simulink model "Excavator_Mevea_BucketDriveline"  (R2026a)
settings: Solver=ode23t  StopTime=29.5  FixedStep=1e-5  MaxStep=Ts  AbsTol=1e-3
PostLoadFcn:
  | set_param(bdroot,'IgnoredZcDiagnostic','none');
  | Excavator_Test_Scenario_Select('loadedBucketDigCycle');
  | Excavator_Mevea_params
StartFcn:
  | tic
StopFcn:
  | elapsedSimTime = toc;
  | disp(['Elapsed Sim Time = ' num2str(elapsedSimTime)]);
model workspace: external: MAT-File ExcavatorAssemblyDataStruct.mat (data not in the file)
undefined symbols (not defined in the file or in its folder): AToBRegOrificeVector, AToTOrificeVector, BiPOrificeVector, BoomC, boomHEArea, boomREArea, boomUpMaxQ, boomValve, BToTOrificeVector, BucketC, bucketCloseMaxQ, bucketOpenMaxQ, BucketR, bucketValve, DiscIntNeverNeededParam, fluids, gravity, K, Lambda, LeftBoomR, maxPumpDisp, minPumpDisp, nominalEngineSpeed, P28Assembly, PToAOrificeVector, PToBOrificeVector, pumpCmdNegRateLimit, pumpCmdPosRateLimit, RightBoomR, StickC, stickInMaxQ, stickOutMaxQ, StickR, stickValve, SwingC, swingDisplacement, swingHighSpeedThreshold, swingMaxQ, SwingR, swingSpeedQGain, swingValve, tau, valveCmdNegRateLimit, valveCmdPosRateLimit, X, x0, Y, Z
libraries: fl_lib x113, SimscapeFluids_lib x78, nesl_utility x61, sm_lib x55, simulink_extras x11, Excavator_Parts_Lib x6, sm_wheel_loader_lib x6, simulink x5, sdl_lib x4, SignalEditorBlockLib x1
(part 5 of 8)

== system Excavator_Mevea_BucketDriveline/Excavator/Machine/Boom Cyl R/BoomRightCyl ==
  BoomRightCyl_primary : sm_lib/Body Elements/File Solid  ExtGeomFileName=BoomRightCyl_Primary.SLDPRT  UnitType=FromFile  ExtGeomFileUnits=m  StepReaderType=HEX  ExportConvexHullGeometry=off  InertiaType=Custom  BasedOnType=DensityFromFile  Density=1000  DensityUnits=kg/m^3  Mass=P28Assembly.bodyGroups(4).subGroups(1).inertialProperties.mass  MassUnits=kg  CenterOfMass=P28Assembly.bodyGroups(4).subGroups(1).inertialProperties.centerOfMass  CenterOfMassUnits=m  MomentsOfInertia=P28Assembly.bodyGroups(4).subGroups(1).inertialProperties.momentsOfInertia  MomentsOfInertiaUnits=kg*m^2  ProductsOfInertia=P28Assembly.bodyGroups(4).subGroups(1).inertialProperties.productsOfInertia  ProductsOfInertiaUnits=kg*m^2  GraphicType=FromGeometry  MarkerShape=Sphere  MarkerSize=10  GraphicVisPropType=SimpleVisualProperties  GraphicDiffuseColor=P28Assembly.bodyGroups(4).subGroups(1).visualProperties.rgb  GraphicOpacity=P28Assembly.bodyGroups(4).subGroups(1).visualProperties.opacity  GraphicSpecularColor=[0.5 0.5 0.5 1.0]  GraphicAmbientColor=[0.15 0.15 0.15 1.0]  GraphicEmissiveColor=[0.0 0.0 0.0 1.0]  GraphicShininess=75  DoExposeReferenceFrame=on  SerializedFrames=<Frames/>
  RT_ChassisToRightBoomCyl : sm_lib/Frames and Transforms/Rigid Transform  RotationMethod=RotationMatrix  FollAlignAxisA=+X  BaseAlignAxisA=+Y  FollAlignAxisB=+Y  BaseAlignAxisB=+Z  RotationStandardAxis=+Z  RotationAngle=0.0  RotationAngleUnits=deg  RotationArbitraryAxis=[0 0 1]  RotationSequenceAxes=FollowerAxes  RotationSequence=XYX  RotationSequenceAngles=[0 0 0]  RotationSequenceAnglesUnits=deg  RotationMatrix=P28Assembly.coordSys(6).transform.rotation  Quaternion=[1 0 0 0]  TranslationMethod=Cartesian  TranslationCartesianOffset=P28Assembly.coordSys(6).transform.translation  TranslationCartesianOffsetUnits=m  TranslationStandardAxis=+Z  TranslationStandardOffset=0  TranslationStandardOffsetUnits=m  TranslationROffset=0  TranslationROffsetUnits=m  TranslationThetaOffset=0  TranslationThetaOffsetUnits=deg  TranslationZOffset=0  TranslationZOffsetUnits=m
  RT_RightBoomCylToRightBoomPiston : sm_lib/Frames and Transforms/Rigid Transform  RotationMethod=RotationMatrix  FollAlignAxisA=+X  BaseAlignAxisA=+Y  FollAlignAxisB=+Y  BaseAlignAxisB=+Z  RotationStandardAxis=+Z  RotationAngle=0.0  RotationAngleUnits=deg  RotationArbitraryAxis=[0 0 1]  RotationSequenceAxes=FollowerAxes  RotationSequence=XYX  RotationSequenceAngles=[0 0 0]  RotationSequenceAnglesUnits=deg  RotationMatrix=P28Assembly.coordSys(19).transform.rotation  Quaternion=[1 0 0 0]  TranslationMethod=Cartesian  TranslationCartesianOffset=P28Assembly.coordSys(19).transform.translation  TranslationCartesianOffsetUnits=m  TranslationStandardAxis=+Z  TranslationStandardOffset=0  TranslationStandardOffsetUnits=m  TranslationROffset=0  TranslationROffsetUnits=m  TranslationThetaOffset=0  TranslationThetaOffsetUnits=deg  TranslationZOffset=0  TranslationZOffsetUnits=m
  B1 : PMIOPort  Side=Left
  F1 : PMIOPort  Port=2  Side=Right
  connections:
  RT_RightBoomCylToRightBoomPiston/RConn1 -- F1/RConn1
  RT_ChassisToRightBoomCyl/RConn1 -- B1/RConn1
  RT_RightBoomCylToRightBoomPiston/LConn1 -- BoomRightCyl_primary/RConn1 -- RT_ChassisToRightBoomCyl/LConn1

== system Excavator_Mevea_BucketDriveline/Excavator/Machine/Boom Cyl R/BoomRightPiston ==
  BoomRightPiston_primary : sm_lib/Body Elements/File Solid  ExtGeomFileName=BoomRightPiston_Primary.SLDPRT  UnitType=FromFile  ExtGeomFileUnits=m  StepReaderType=HEX  ExportConvexHullGeometry=off  InertiaType=Custom  BasedOnType=DensityFromFile  Density=1000  DensityUnits=kg/m^3  Mass=P28Assembly.bodyGroups(5).subGroups(1).inertialProperties.mass  MassUnits=kg  CenterOfMass=P28Assembly.bodyGroups(5).subGroups(1).inertialProperties.centerOfMass  CenterOfMassUnits=m  MomentsOfInertia=P28Assembly.bodyGroups(5).subGroups(1).inertialProperties.momentsOfInertia  MomentsOfInertiaUnits=kg*m^2  ProductsOfInertia=P28Assembly.bodyGroups(5).subGroups(1).inertialProperties.productsOfInertia  ProductsOfInertiaUnits=kg*m^2  GraphicType=FromGeometry  MarkerShape=Sphere  MarkerSize=10  GraphicVisPropType=SimpleVisualProperties  GraphicDiffuseColor=P28Assembly.bodyGroups(5).subGroups(1).visualProperties.rgb  GraphicOpacity=P28Assembly.bodyGroups(5).subGroups(1).visualProperties.opacity  GraphicSpecularColor=[0.5 0.5 0.5 1.0]  GraphicAmbientColor=[0.15 0.15 0.15 1.0]  GraphicEmissiveColor=[0.0 0.0 0.0 1.0]  GraphicShininess=75  DoExposeReferenceFrame=on  SerializedFrames=<Frames/>
  RT_BoomToRightBoomPiston : sm_lib/Frames and Transforms/Rigid Transform  RotationMethod=RotationMatrix  FollAlignAxisA=+X  BaseAlignAxisA=+Y  FollAlignAxisB=+Y  BaseAlignAxisB=+Z  RotationStandardAxis=+Z  RotationAngle=0.0  RotationAngleUnits=deg  RotationArbitraryAxis=[0 0 1]  RotationSequenceAxes=FollowerAxes  RotationSequence=XYX  RotationSequenceAngles=[0 0 0]  RotationSequenceAnglesUnits=deg  RotationMatrix=P28Assembly.coordSys(7).transform.rotation  Quaternion=[1 0 0 0]  TranslationMethod=Cartesian  TranslationCartesianOffset=P28Assembly.coordSys(7).transform.translation  TranslationCartesianOffsetUnits=m  TranslationStandardAxis=+Z  TranslationStandardOffset=0  TranslationStandardOffsetUnits=m  TranslationROffset=0  TranslationROffsetUnits=m  TranslationThetaOffset=0  TranslationThetaOffsetUnits=deg  TranslationZOffset=0  TranslationZOffsetUnits=m
  RT_RightBoomCylToRightBoomPiston : sm_lib/Frames and Transforms/Rigid Transform  RotationMethod=RotationMatrix  FollAlignAxisA=+X  BaseAlignAxisA=+Y  FollAlignAxisB=+Y  BaseAlignAxisB=+Z  RotationStandardAxis=+Z  RotationAngle=0.0  RotationAngleUnits=deg  RotationArbitraryAxis=[0 0 1]  RotationSequenceAxes=FollowerAxes  RotationSequence=XYX  RotationSequenceAngles=[0 0 0]  RotationSequenceAnglesUnits=deg  RotationMatrix=P28Assembly.coordSys(19).transform.rotation  Quaternion=[1 0 0 0]  TranslationMethod=Cartesian  TranslationCartesianOffset=P28Assembly.coordSys(19).transform.translation  TranslationCartesianOffsetUnits=m  TranslationStandardAxis=+Z  TranslationStandardOffset=0  TranslationStandardOffsetUnits=m  TranslationROffset=0  TranslationROffsetUnits=m  TranslationThetaOffset=0  TranslationThetaOffsetUnits=deg  TranslationZOffset=0  TranslationZOffsetUnits=m
  B1 : PMIOPort  Side=Right
  B2 : PMIOPort  Port=2  Side=Left
  connections:
  RT_RightBoomCylToRightBoomPiston/RConn1 -- B2/RConn1
  RT_BoomToRightBoomPiston/RConn1 -- B1/RConn1
  RT_RightBoomCylToRightBoomPiston/LConn1 -- BoomRightPiston_primary/RConn1 -- RT_BoomToRightBoomPiston/LConn1

== system Excavator_Mevea_BucketDriveline/Excavator/Machine/Boom Cyl R/RightBoomCylToRightBoomPiston ==
  RightBoomCylToRightBoomPiston : sm_lib/Joints/Cylindrical Joint  JointMode=Normal  CompositeWrenchDir=FollowerOnBase  CompositeWrenchFrame=BaseFrame  SenseConstraintForce=off  SenseConstraintTorque=off  SenseTotalForce=off  SenseTotalTorque=off  RzPositionTargetSpecify=off  RzPositionTargetPriority=High  RzPositionTargetValue=0  RzPositionTargetValueUnits=deg  RzVelocityTargetSpecify=off  RzVelocityTargetPriority=High  RzVelocityTargetValue=0  RzVelocityTargetValueUnits=deg/s  RzEquilibriumPosition=0  RzEquilibriumPositionUnits=deg  RzSpringStiffness=0  RzSpringStiffnessUnits=N*m/deg  RzDampingCoefficient=0  RzDampingCoefficientUnits=N*m/(deg/s)  RzLowerLimitSpecify=off  RzLowerLimitBound=-90  RzLowerLimitBoundUnits=deg  RzLowerLimitStiffness=1e4  RzLowerLimitStiffnessUnits=N*m/deg  RzLowerLimitDamping=10  RzLowerLimitDampingUnits=N*m/(deg/s)  RzLowerLimitTransitionRegionWidth=0.1  RzLowerLimitTransitionRegionWidthUnits=deg  RzUpperLimitSpecify=off  RzUpperLimitBound=90  RzUpperLimitBoundUnits=deg  RzUpperLimitStiffness=1e4  RzUpperLimitStiffnessUnits=N*m/deg  RzUpperLimitDamping=10  RzUpperLimitDampingUnits=N*m/(deg/s)  RzUpperLimitTransitionRegionWidth=0.1  RzUpperLimitTransitionRegionWidthUnits=deg  RzTorqueActuationMode=NoTorque  RzMotionActuationMode=ComputedMotion  RzSensePosition=off  RzSenseVelocity=off  RzSenseAcceleration=off  RzSenseTorqueForce=off  RzSenseLowerLimitTorqueForce=off  RzSenseUpperLimitTorqueForce=off  PzPositionTargetSpecify=on  PzPositionTargetPriority=High  PzPositionTargetValue=initBoomPistonPos  PzPositionTargetValueUnits=mm  PzVelocityTargetSpecify=off  PzVelocityTargetPriority=High  PzVelocityTargetValue=0  PzVelocityTargetValueUnits=m/s  PzEquilibriumPosition=0  PzEquilibriumPositionUnits=m  PzSpringStiffness=0  PzSpringStiffnessUnits=N/m  PzDampingCoefficient=0  PzDampingCoefficientUnits=N/(m/s)  PzLowerLimitSpecify=off  PzLowerLimitBound=-1  PzLowerLimitBoundUnits=m  PzLowerLimitStiffness=1e6  PzLowerLimitStiffnessUnits=N/m  PzLowerLimitDamping=1e3  PzLowerLimitDampingUnits=N/(m/s)  PzLowerLimitTransitionRegionWidth=1e-4  PzLowerLimitTransitionRegionWidthUnits=m  PzUpperLimitSpecify=off  PzUpperLimitBound=1  PzUpperLimitBoundUnits=m  PzUpperLimitStiffness=1e6  PzUpperLimitStiffnessUnits=N/m  PzUpperLimitDamping=1e3  PzUpperLimitDampingUnits=N/(m/s)  PzUpperLimitTransitionRegionWidth=1e-4  PzUpperLimitTransitionRegionWidthUnits=m  PzTorqueActuationMode=InputTorque  PzMotionActuationMode=ComputedMotion  PzSensePosition=off  PzSenseVelocity=on  PzSenseAcceleration=off  PzSenseTorqueForce=off  PzSenseLowerLimitTorqueForce=off  PzSenseUpperLimitTorqueForce=off
  Simscape Bus : SimscapeBus  HierarchyStrings=BoomC;RightBoomR
  Translational Multibody Interface : fl_lib/Mechanical/Multibody Interfaces/Translational Multibody Interface
  BoomHydToMech : PMIOPort  Side=Left
  B : PMIOPort  Port=2  Side=Left
  F : PMIOPort  Port=3  Side=Right
  connections:
  RightBoomCylToRightBoomPiston/RConn1 -- F/RConn1
  RightBoomCylToRightBoomPiston/LConn1 -- B/RConn1
  Translational Multibody Interface/LConn1 -- RightBoomCylToRightBoomPiston/LConn2
  Translational Multibody Interface/RConn1 -- RightBoomCylToRightBoomPiston/RConn2
  Simscape Bus/RConn1 -- BoomHydToMech/RConn1
  Simscape Bus/LConn1 -- Translational Multibody Interface/LConn2
  Simscape Bus/LConn2 -- Translational Multibody Interface/RConn2

== system Excavator_Mevea_BucketDriveline/Excavator/Machine/Bucket Cyl/BucketCyl ==
  BucketCyl_primary : sm_lib/Body Elements/File Solid  ExtGeomFileName=BucketCyl_Primary.SLDPRT  UnitType=FromFile  ExtGeomFileUnits=m  StepReaderType=HEX  ExportConvexHullGeometry=off  InertiaType=Custom  BasedOnType=DensityFromFile  Density=1000  DensityUnits=kg/m^3  Mass=P28Assembly.bodyGroups(10).subGroups(1).inertialProperties.mass  MassUnits=kg  CenterOfMass=P28Assembly.bodyGroups(10).subGroups(1).inertialProperties.centerOfMass  CenterOfMassUnits=m  MomentsOfInertia=P28Assembly.bodyGroups(10).subGroups(1).inertialProperties.momentsOfInertia  MomentsOfInertiaUnits=kg*m^2  ProductsOfInertia=P28Assembly.bodyGroups(10).subGroups(1).inertialProperties.productsOfInertia  ProductsOfInertiaUnits=kg*m^2  GraphicType=FromGeometry  MarkerShape=Sphere  MarkerSize=10  GraphicVisPropType=SimpleVisualProperties  GraphicDiffuseColor=P28Assembly.bodyGroups(10).subGroups(1).visualProperties.rgb  GraphicOpacity=P28Assembly.bodyGroups(10).subGroups(1).visualProperties.opacity  GraphicSpecularColor=[0.5 0.5 0.5 1.0]  GraphicAmbientColor=[0.15 0.15 0.15 1.0]  GraphicEmissiveColor=[0.0 0.0 0.0 1.0]  GraphicShininess=75  DoExposeReferenceFrame=on  SerializedFrames=<Frames/>
  RT_BucketCylToBucketPiston : sm_lib/Frames and Transforms/Rigid Transform  RotationMethod=RotationMatrix  FollAlignAxisA=+X  BaseAlignAxisA=+Y  FollAlignAxisB=+Y  BaseAlignAxisB=+Z  RotationStandardAxis=+Z  RotationAngle=0.0  RotationAngleUnits=deg  RotationArbitraryAxis=[0 0 1]  RotationSequenceAxes=FollowerAxes  RotationSequence=XYX  RotationSequenceAngles=[0 0 0]  RotationSequenceAnglesUnits=deg  RotationMatrix=P28Assembly.coordSys(21).transform.rotation  Quaternion=[1 0 0 0]  TranslationMethod=Cartesian  TranslationCartesianOffset=P28Assembly.coordSys(21).transform.translation  TranslationCartesianOffsetUnits=m  TranslationStandardAxis=+Z  TranslationStandardOffset=0  TranslationStandardOffsetUnits=m  TranslationROffset=0  TranslationROffsetUnits=m  TranslationThetaOffset=0  TranslationThetaOffsetUnits=deg  TranslationZOffset=0  TranslationZOffsetUnits=m
  RT_StickToBucketCyl : sm_lib/Frames and Transforms/Rigid Transform  RotationMethod=RotationMatrix  FollAlignAxisA=+X  BaseAlignAxisA=+Y  FollAlignAxisB=+Y  BaseAlignAxisB=+Z  RotationStandardAxis=+Z  RotationAngle=0.0  RotationAngleUnits=deg  RotationArbitraryAxis=[0 0 1]  RotationSequenceAxes=FollowerAxes  RotationSequence=XYX  RotationSequenceAngles=[0 0 0]  RotationSequenceAnglesUnits=deg  RotationMatrix=P28Assembly.coordSys(11).transform.rotation  Quaternion=[1 0 0 0]  TranslationMethod=Cartesian  TranslationCartesianOffset=P28Assembly.coordSys(11).transform.translation  TranslationCartesianOffsetUnits=m  TranslationStandardAxis=+Z  TranslationStandardOffset=0  TranslationStandardOffsetUnits=m  TranslationROffset=0  TranslationROffsetUnits=m  TranslationThetaOffset=0  TranslationThetaOffsetUnits=deg  TranslationZOffset=0  TranslationZOffsetUnits=m
  B1 : PMIOPort  Side=Left
  F1 : PMIOPort  Port=2  Side=Right
  connections:
  RT_StickToBucketCyl/LConn1 -- BucketCyl_primary/RConn1 -- RT_BucketCylToBucketPiston/LConn1
  RT_StickToBucketCyl/RConn1 -- B1/RConn1
  RT_BucketCylToBucketPiston/RConn1 -- F1/RConn1

== system Excavator_Mevea_BucketDriveline/Excavator/Machine/Bucket Cyl/BucketCylToBucketPiston ==
  BucketCylToBucketPiston : sm_lib/Joints/Cylindrical Joint  JointMode=Normal  CompositeWrenchDir=FollowerOnBase  CompositeWrenchFrame=BaseFrame  SenseConstraintForce=off  SenseConstraintTorque=off  SenseTotalForce=off  SenseTotalTorque=off  RzPositionTargetSpecify=off  RzPositionTargetPriority=High  RzPositionTargetValue=0  RzPositionTargetValueUnits=deg  RzVelocityTargetSpecify=off  RzVelocityTargetPriority=High  RzVelocityTargetValue=0  RzVelocityTargetValueUnits=deg/s  RzEquilibriumPosition=0  RzEquilibriumPositionUnits=deg  RzSpringStiffness=0  RzSpringStiffnessUnits=N*m/deg  RzDampingCoefficient=0  RzDampingCoefficientUnits=N*m/(deg/s)  RzLowerLimitSpecify=off  RzLowerLimitBound=-90  RzLowerLimitBoundUnits=deg  RzLowerLimitStiffness=1e4  RzLowerLimitStiffnessUnits=N*m/deg  RzLowerLimitDamping=10  RzLowerLimitDampingUnits=N*m/(deg/s)  RzLowerLimitTransitionRegionWidth=0.1  RzLowerLimitTransitionRegionWidthUnits=deg  RzUpperLimitSpecify=off  RzUpperLimitBound=90  RzUpperLimitBoundUnits=deg  RzUpperLimitStiffness=1e4  RzUpperLimitStiffnessUnits=N*m/deg  RzUpperLimitDamping=10  RzUpperLimitDampingUnits=N*m/(deg/s)  RzUpperLimitTransitionRegionWidth=0.1  RzUpperLimitTransitionRegionWidthUnits=deg  RzTorqueActuationMode=NoTorque  RzMotionActuationMode=ComputedMotion  RzSensePosition=off  RzSenseVelocity=off  RzSenseAcceleration=off  RzSenseTorqueForce=off  RzSenseLowerLimitTorqueForce=off  RzSenseUpperLimitTorqueForce=off  PzPositionTargetSpecify=on  PzPositionTargetPriority=High  PzPositionTargetValue=initBucketPistonPos  PzPositionTargetValueUnits=mm  PzVelocityTargetSpecify=off  PzVelocityTargetPriority=High  PzVelocityTargetValue=0  PzVelocityTargetValueUnits=m/s  PzEquilibriumPosition=0  PzEquilibriumPositionUnits=m  PzSpringStiffness=0  PzSpringStiffnessUnits=N/m  PzDampingCoefficient=0  PzDampingCoefficientUnits=N/(m/s)  PzLowerLimitSpecify=off  PzLowerLimitBound=-1  PzLowerLimitBoundUnits=m  PzLowerLimitStiffness=1e6  PzLowerLimitStiffnessUnits=N/m  PzLowerLimitDamping=1e3  PzLowerLimitDampingUnits=N/(m/s)  PzLowerLimitTransitionRegionWidth=1e-4  PzLowerLimitTransitionRegionWidthUnits=m  PzUpperLimitSpecify=off  PzUpperLimitBound=1  PzUpperLimitBoundUnits=m  PzUpperLimitStiffness=1e6  PzUpperLimitStiffnessUnits=N/m  PzUpperLimitDamping=1e3  PzUpperLimitDampingUnits=N/(m/s)  PzUpperLimitTransitionRegionWidth=1e-4  PzUpperLimitTransitionRegionWidthUnits=m  PzTorqueActuationMode=InputTorque  PzMotionActuationMode=ComputedMotion  PzSensePosition=off  PzSenseVelocity=on  PzSenseAcceleration=off  PzSenseTorqueForce=off  PzSenseLowerLimitTorqueForce=off  PzSenseUpperLimitTorqueForce=off
  Simscape Bus : SimscapeBus  HierarchyStrings=BucketC;BucketR
  Translational Multibody Interface : fl_lib/Mechanical/Multibody Interfaces/Translational Multibody Interface
  B : PMIOPort  Side=Left
  F : PMIOPort  Port=2  Side=Right
  BucketHydToMech : PMIOPort  Port=3  Side=Left
  connections:
  B/RConn1 -- BucketCylToBucketPiston/LConn1
  Simscape Bus/RConn1 -- BucketHydToMech/RConn1
  Translational Multibody Interface/LConn2 -- Simscape Bus/LConn1
  Simscape Bus/LConn2 -- Translational Multibody Interface/RConn2
  Translational Multibody Interface/RConn1 -- BucketCylToBucketPiston/RConn2
  Translational Multibody Interface/LConn1 -- BucketCylToBucketPiston/LConn2
  BucketCylToBucketPiston/RConn1 -- F/RConn1

== system Excavator_Mevea_BucketDriveline/Excavator/Machine/Bucket Cyl/BucketPiston ==
  BucketPiston_primary : sm_lib/Body Elements/File Solid  ExtGeomFileName=BucketPiston_Primary.SLDPRT  UnitType=FromFile  ExtGeomFileUnits=m  StepReaderType=HEX  ExportConvexHullGeometry=off  InertiaType=Custom  BasedOnType=DensityFromFile  Density=1000  DensityUnits=kg/m^3  Mass=P28Assembly.bodyGroups(11).subGroups(1).inertialProperties.mass  MassUnits=kg  CenterOfMass=P28Assembly.bodyGroups(11).subGroups(1).inertialProperties.centerOfMass  CenterOfMassUnits=m  MomentsOfInertia=P28Assembly.bodyGroups(11).subGroups(1).inertialProperties.momentsOfInertia  MomentsOfInertiaUnits=kg*m^2  ProductsOfInertia=P28Assembly.bodyGroups(11).subGroups(1).inertialProperties.productsOfInertia  ProductsOfInertiaUnits=kg*m^2  GraphicType=FromGeometry  MarkerShape=Sphere  MarkerSize=10  GraphicVisPropType=SimpleVisualProperties  GraphicDiffuseColor=P28Assembly.bodyGroups(11).subGroups(1).visualProperties.rgb  GraphicOpacity=P28Assembly.bodyGroups(11).subGroups(1).visualProperties.opacity  GraphicSpecularColor=[0.5 0.5 0.5 1.0]  GraphicAmbientColor=[0.15 0.15 0.15 1.0]  GraphicEmissiveColor=[0.0 0.0 0.0 1.0]  GraphicShininess=75  DoExposeReferenceFrame=on  SerializedFrames=<Frames/>
  RT_BucketCylToBucketPiston : sm_lib/Frames and Transforms/Rigid Transform  RotationMethod=RotationMatrix  FollAlignAxisA=+X  BaseAlignAxisA=+Y  FollAlignAxisB=+Y  BaseAlignAxisB=+Z  RotationStandardAxis=+Z  RotationAngle=0.0  RotationAngleUnits=deg  RotationArbitraryAxis=[0 0 1]  RotationSequenceAxes=FollowerAxes  RotationSequence=XYX  RotationSequenceAngles=[0 0 0]  RotationSequenceAnglesUnits=deg  RotationMatrix=P28Assembly.coordSys(21).transform.rotation  Quaternion=[1 0 0 0]  TranslationMethod=Cartesian  TranslationCartesianOffset=P28Assembly.coordSys(21).transform.translation  TranslationCartesianOffsetUnits=m  TranslationStandardAxis=+Z  TranslationStandardOffset=0  TranslationStandardOffsetUnits=m  TranslationROffset=0  TranslationROffsetUnits=m  TranslationThetaOffset=0  TranslationThetaOffsetUnits=deg  TranslationZOffset=0  TranslationZOffsetUnits=m
  RT_BucketPistonToBucketLink : sm_lib/Frames and Transforms/Rigid Transform  RotationMethod=RotationMatrix  FollAlignAxisA=+X  BaseAlignAxisA=+Y  FollAlignAxisB=+Y  BaseAlignAxisB=+Z  RotationStandardAxis=+Z  RotationAngle=0.0  RotationAngleUnits=deg  RotationArbitraryAxis=[0 0 1]  RotationSequenceAxes=FollowerAxes  RotationSequence=XYX  RotationSequenceAngles=[0 0 0]  RotationSequenceAnglesUnits=deg  RotationMatrix=P28Assembly.coordSys(12).transform.rotation  Quaternion=[1 0 0 0]  TranslationMethod=Cartesian  TranslationCartesianOffset=P28Assembly.coordSys(12).transform.translation  TranslationCartesianOffsetUnits=m  TranslationStandardAxis=+Z  TranslationStandardOffset=0  TranslationStandardOffsetUnits=m  TranslationROffset=0  TranslationROffsetUnits=m  TranslationThetaOffset=0  TranslationThetaOffsetUnits=deg  TranslationZOffset=0  TranslationZOffsetUnits=m
  B1 : PMIOPort  Side=Left
  F1 : PMIOPort  Port=2  Side=Right
  connections:
  BucketPiston_primary/RConn1 -- RT_BucketCylToBucketPiston/LConn1 -- RT_BucketPistonToBucketLink/LConn1
  RT_BucketCylToBucketPiston/RConn1 -- B1/RConn1
  RT_BucketPistonToBucketLink/RConn1 -- F1/RConn1

== system Excavator_Mevea_BucketDriveline/Excavator/Machine/Mevea/FMU ==
  mBucket : Inport
  mChassis : Inport  Port=2
  mRight : Inport  Port=3
  mLeft : Inport  Port=4
  Brk : Inport  Port=5
  Demux : Demux  Outputs=13
  Demux11 : Demux  Outputs=13
  FMU : FMU  FMUName=MeveaLargeExcavatorTCFMUCSControl.fmu  FMUMode=CoSimulation  FMUInitializeEnumObject=off  FMUCachedDialogLayout="{\"Geometry\":[2658,147,869,770],\"ParameterColumnsWidthConfig\":\"{\\\"columns\\\":[{\\\"name\\\":\\\"Parameter\\\",\\\"width\\\":223},{\\\"name\\\":\\\"Value\\\",\\\"width\\\":194},{\\\"name\\\":\\\"Unit\\\",\\\"width\\\":186},{\\\"name\\\":\\\"Description\\\",\\\"width\\\":229}]}\",\"InputColumnsWidthConfig\":\"{\\\"columns\\\":[{\\\"name\\\":\\\"Name\\\",\\\"width\\\":189},{\\\"name\\\":\\\"Visibility\\\",\\\"width\\\":60},{\\\"name\\\":\\\"Start\\\",\\\"width\\\":181},{\\\"name\\\":\\\"Unit\\\",\\\"width\\\":177},{\\\"name\\\":\\\"Type Object\\\",\\\"width\\\":221}]}\",\"OutputColumnsWidthConfig\":[]}"  DV_RollerHeigth=-0.73  DV_RollerDistance=0.35  DV_Roller1_Posx=2.1  DV_Roller2_Posx=1.75  DV_Roller3_Posx=1.4  DV_Roller4_Posx=1.05  DV_Roller5_Posx=0.7  DV_Roller6_Posx=0.35  DV_Roller7_Posx=0  DV_Roller8_Posx=-0.35  DV_Roller9_Posx=-0.70  DV_Roller10_Posx=-1.05  DV_Roller11_Posx=-1.4  DV_Roller12_Posx=-1.75  DV_Roller13_Posx=-2.1  DV_SprocketRadius=0.50  DV_RollerRadius=0.15  DV_RollerDamping=3  DV_SprocketDamping=5  DV_SprocketMass=615  socketPort=int32(5111)  useHeadlessSolver=int32(0)  activateAssemblies="\"\""  deactivateAssemblies="\"\""  solverIPaddress='127.0.0.1'  mask(MeveaExcavatorExternalCSControl [Co-Simulation, v2.0]){}
      mask Display:
      | disp('MeveaExcavatorExternalCSControl');
      | port_label('output',1,'SO_BucketForce_X');
      | port_label('output',2,'SO_BucketForce_Y');
      | port_label('output',3,'SO_BucketForce_Z');
      | port_label('output',4,'SO_BucketTorque_X');
      | port_label('output',5,'SO_BucketTorque_Y');
      | port_label('output',6,'SO_BucketTorque_Z');
      | port_label('output',7,'SO_UndercarriageForce_X');
      | port_label('output',8,'SO_UndercarriageForce_Y');
      | port_label('output',9,'SO_UndercarriageForce_Z');
      | port_label('output',10,'SO_UndercarriageTorque_X');
      | port_label('output',11,'SO_UndercarriageTorque_Y');
      | port_label('output',12,'SO_UndercarriageTorque_Z');
      | port_label('output',13,'SO_LeftCrawler_w');
      | port_label('output',14,'SO_RightCrawler_w');
      | port_label('input',1,'SI_BucketVelocity_X');
      | port_label('input',2,'SI_BucketVelocity_Y');
      | port_label('input',3,'SI_BucketVelocity_Z');
      | port_label('input',4,'SI_BucketOmega_X');
      | port_label('input',5,'SI_BucketOmega_Y');
      | port_label('input',6,'SI_BucketOmega_Z');
      | port_label('input',7,'SI_BucketPosition_X');
      | port_label('input',8,'SI_BucketPosition_Y');
      | port_label('input',9,'SI_BucketPosition_Z');
      | port_label('input',10,'SI_BucketQuat_w');
      | port_label('input',11,'SI_BucketQuat_ux');
      | port_label('input',12,'SI_BucketQuat_uy');
      | port_label('input',13,'SI_BucketQuat_uz');
      | port_label('input',14,'SI_UndercarriageVelocity_X');
      | port_label('input',15,'SI_UndercarriageVelocity_Y');
      | port_label('input',16,'SI_UndercarriageVelocity_Z');
      | port_label('input',17,'SI_UndercarriageOmega_X');
      | port_label('input',18,'SI_UndercarriageOmega_Y');
      | port_label('input',19,'SI_UndercarriageOmega_Z');
      | port_label('input',20,'SI_UndercarriagePosition_X');
      | port_label('input',21,'SI_UndercarriagePosition_Y');
      | port_label('input',22,'SI_UndercarriagePosition_Z');
      | port_label('input',23,'SI_UndercarriageQuat_w');
      | port_label('input',24,'SI_UndercarriageQuat_ux');
      | port_label('input',25,'SI_UndercarriageQuat_uy');
      | port_label('input',26,'SI_UndercarriageQuat_uz');
      | port_label('input',27,'SI_LeftCrawler_T');
      | port_label('input',28,'SI_RightCrawler_T');
      | port_label('input',29,'SI_CrawlerBrake');
  Mux5 : Mux  Inputs=6
  Mux6 : Mux  Inputs=6
  fBucket : Outport
  fChassis : Outport  Port=2
  tRight : Outport  Port=3
  tLeft : Outport  Port=4
  wires:
  mChassis/1 -> Demux11/1
  Demux11/13 -> FMU/26
  FMU/10 -> Mux5/4
  Demux/2 -> FMU/2
  Brk/1 -> FMU/29
  FMU/13 -> tRight/1
  Demux11/12 -> FMU/25
  Demux/1 -> FMU/1
  FMU/8 -> Mux5/2
  Demux11/10 -> FMU/23
  FMU/4 -> Mux6/4
  Demux/9 -> FMU/9
  Demux11/11 -> FMU/24
  Demux/5 -> FMU/5
  FMU/2 -> Mux6/2
  Demux11/7 -> FMU/20
  FMU/5 -> Mux6/5
  Demux/6 -> FMU/6
  FMU/3 -> Mux6/3
  Demux/8 -> FMU/8
  Demux11/1 -> FMU/14
  FMU/9 -> Mux5/3
  FMU/7 -> Mux5/1
  Demux11/5 -> FMU/18
  Demux11/2 -> FMU/15
  Demux11/3 -> FMU/16
  Demux/13 -> FMU/13
  Demux11/6 -> FMU/19
  Demux11/4 -> FMU/17
  FMU/1 -> Mux6/1
  Demux11/8 -> FMU/21
  mLeft/1 -> FMU/27
  mRight/1 -> FMU/28
  Demux11/9 -> FMU/22
  Demux/10 -> FMU/10
  FMU/12 -> Mux5/6
  FMU/6 -> Mux6/6
  FMU/11 -> Mux5/5
  FMU/14 -> tLeft/1
  Demux/11 -> FMU/11
  Demux/12 -> FMU/12
  Demux/7 -> FMU/7
  Demux/4 -> FMU/4
  Demux/3 -> FMU/3
  Mux6/1 -> fBucket/1
  mBucket/1 -> Demux/1
  Mux5/1 -> fChassis/1

== system Excavator_Mevea_BucketDriveline/Excavator/Machine/Mevea/Forces Bucket ==
  ft : Inport
  Demux10 : Demux  Outputs=6
  First Order Hold : FirstOrderHold  ErrorTolerance=inf  AllowContinuousInput=on
  First Order Hold1 : FirstOrderHold  ErrorTolerance=inf  AllowContinuousInput=on
  Mux : Mux  Inputs=3
  Mux1 : Mux  Inputs=3
  Simulink-PS Converter2 : nesl_utility/Simulink-PS Converter  PhysicalDomain=network_engine_domain  SubClassName=ps_input  LeftPortType=input  RightPortType=output  PseudoPeriodic=off  Frequencies=[]  NoiseDistribution=none  NoiseParameters=[]  Unit=N  AffineConversion=off  FilteringAndDerivatives=provide  SimscapeFilterOrder=1  InputFilterTimeConstant=0.001  UdotUserProvided=0
  Simulink-PS Converter3 : nesl_utility/Simulink-PS Converter  PhysicalDomain=network_engine_domain  SubClassName=ps_input  LeftPortType=input  RightPortType=output  PseudoPeriodic=off  Frequencies=[]  NoiseDistribution=none  NoiseParameters=[]  Unit=N*m  AffineConversion=off  FilteringAndDerivatives=provide  SimscapeFilterOrder=1  InputFilterTimeConstant=0.001  UdotUserProvided=0
  frc : PMIOPort  Side=Right
  trq : PMIOPort  Port=2  Side=Right
  wires:
  Mux/1 -> First Order Hold/1
  Demux10/3 -> Mux/3
  First Order Hold1/1 -> Simulink-PS Converter3/1
  Demux10/6 -> Mux1/3
  Demux10/2 -> Mux/2
  Demux10/5 -> Mux1/2
  Mux1/1 -> First Order Hold1/1
  First Order Hold/1 -> Simulink-PS Converter2/1
  Demux10/1 -> Mux/1
  Demux10/4 -> Mux1/1
  ft/1 -> Demux10/1
  connections:
  Simulink-PS Converter2/RConn1 -- frc/RConn1
  Simulink-PS Converter3/RConn1 -- trq/RConn1

== system Excavator_Mevea_BucketDriveline/Excavator/Machine/Mevea/Forces Chassis ==
  ft : Inport
  Demux9 : Demux  Outputs=6
  First Order Hold2 : FirstOrderHold  ErrorTolerance=inf  AllowContinuousInput=on
  First Order Hold3 : FirstOrderHold  ErrorTolerance=inf  AllowContinuousInput=on
  Mux2 : Mux  Inputs=3
  Mux3 : Mux  Inputs=3
  Simulink-PS Converter1 : nesl_utility/Simulink-PS Converter  PhysicalDomain=network_engine_domain  SubClassName=ps_input  LeftPortType=input  RightPortType=output  PseudoPeriodic=off  Frequencies=[]  NoiseDistribution=none  NoiseParameters=[]  Unit=N  AffineConversion=off  FilteringAndDerivatives=provide  SimscapeFilterOrder=1  InputFilterTimeConstant=0.001  UdotUserProvided=0
  Simulink-PS Converter4 : nesl_utility/Simulink-PS Converter  PhysicalDomain=network_engine_domain  SubClassName=ps_input  LeftPortType=input  RightPortType=output  PseudoPeriodic=off  Frequencies=[]  NoiseDistribution=none  NoiseParameters=[]  Unit=N*m  AffineConversion=off  FilteringAndDerivatives=provide  SimscapeFilterOrder=1  InputFilterTimeConstant=0.001  UdotUserProvided=0
  frc : PMIOPort  Side=Right
  trq : PMIOPort  Port=2  Side=Right
  wires:
  Demux9/3 -> Mux2/3
  Demux9/6 -> Mux3/3
  Mux3/1 -> First Order Hold3/1
  Demux9/4 -> Mux3/1
  ft/1 -> Demux9/1
  Demux9/2 -> Mux2/2
  Mux2/1 -> First Order Hold2/1
  First Order Hold2/1 -> Simulink-PS Converter1/1
  Demux9/1 -> Mux2/1
  First Order Hold3/1 -> Simulink-PS Converter4/1
  Demux9/5 -> Mux3/2
  connections:
  Simulink-PS Converter4/RConn1 -- trq/RConn1
  Simulink-PS Converter1/RConn1 -- frc/RConn1

== system Excavator_Mevea_BucketDriveline/Excavator/Machine/Mevea/Interface CrawlerL ==
  note: Uncomment rate transition
      | blocks if one or both networks
      | are running fixed step.
  spd : Inport
  First Order Hold3 : FirstOrderHold  ErrorTolerance=inf  AllowContinuousInput=on
  Gain : Gain
  Gain1 : Gain  Gain=-1
  Ideal Rotational Motion Sensor : fl_lib/Mechanical/Mechanical Sensors/Ideal Rotational Motion Sensor  reference=foundation.enum.MeasurementReference.absolute  acceleration_port=false  velocity_port=true  position_port=false  wrap_angle=false  offset=0 rad
  Mux : Mux  Inputs=2
  PS-Simulink Converter : nesl_utility/PS-Simulink Converter  PhysicalDomain=network_engine_domain  SubClassName=ps_output  LeftPortType=input  RightPortType=output  PseudoPeriodic=off  Frequencies=[]  VectorFormat=inherit  Unit=rad/s  AffineConversion=off
  Port 1 Interface : Subsystem  mask(Network Coupler (Flexible Shaft) Port 1 Interface){interfaceModel=an actual shaft compliance, k=2500, lambda=200, samplingType=Variable step at ports 1 and 2, ts=0.002, h1=0.001, h2=0.01, predictionDiscreteToContinuous=off, smoothingContinuousToDiscrete=off, predictionSlowToFast=off, smoothingFastToSlow=off, nSmooth=1, tsSmoothing=0.01, J1=1, J2=1, tsRecommended=NaN, hRecommended=2.7764e-05, kDerived=2500, lambdaDerived=200, tsMax=0.012494, through0=0}
      mask prompts: interfaceModel "physmod:simscape:couplers:SimscapeNetworkCouplersLib:SeparateUsing_MP"; k "physmod:simscape:couplers:SimscapeNetworkCouplersLib:ShaftStiffnessNmrad_MP"; lambda "physmod:simscape:couplers:SimscapeNetworkCouplersLib:ShaftDampingNmrads_MP"; samplingType "physmod:simscape:couplers:SimscapeNetworkCouplersLib:SamplingType_MP"; ts "physmod:simscape:couplers:SimscapeNetworkCouplersLib:SeparatorTimeConstants_MP"; h1 "physmod:simscape:couplers:SimscapeNetworkCouplersLib:Port1NetworkDiscreteSampleTimes_MP"; h2 "physmod:simscape:couplers:SimscapeNetworkCouplersLib:Port2NetworkDiscreteSampleTimes_MP"; predictionDiscreteToContinuous "physmod:simscape:couplers:SimscapeNetworkCouplersLib:UsePredictionWhenConnectingFixedStepToVariableStep_MP"; smoothingContinuousToDiscrete "physmod:simscape:couplers:SimscapeNetworkCouplersLib:UseSmoothingWhenConnectingVariableStepToFixedStep_MP"; predictionSlowToFast "physmod:simscape:couplers:SimscapeNetworkCouplersLib:UsePredictionWhenConnectingSlowToFastSampleTimes_MP"; smoothingFastToSlow "physmod:simscape:couplers:SimscapeNetworkCouplersLib:UseSmoothingWhenConnectingFastToSlowSampleTimes_MP"; nSmooth "physmod:simscape:couplers:SimscapeNetworkCouplersLib:NumberOfSamplesOverWhichToSmooth_MP"; tsSmoothing "physmod:simscape:couplers:SimscapeNetworkCouplersLib:SmoothingTimeConstants_MP"; J1 "physmod:simscape:couplers:SimscapeNetworkCouplersLib:ApproximateInertiaAtPort1kgm2_MP"; J2 "physmod:simscape:couplers:SimscapeNetworkCouplersLib:ApproximateInertiaAtPort2kgm2_MP"; tsRecommended "physmod:simscape:couplers:SimscapeNetworkCouplersLib:RecommendedMaxFilterTimeConstants_MP"; hRecommended "physmod:simscape:couplers:SimscapeNetworkCouplersLib:RecommendedMaxDiscreteSampleTimes_MP"; kDerived "physmod:simscape:couplers:SimscapeNetworkCouplersLib:CalculatedShaftStiffnessNmrad_MP"; lambdaDerived "physmod:simscape:couplers:SimscapeNetworkCouplersLib:CalculatedShaftDampingNmrads_MP"; tsMax "physmod:simscape:couplers:SimscapeNetworkCouplersLib:CalculatedFastestTrackableTimeConstants_MP"; through0 "physmod:simscape:couplers:SimscapeNetworkCouplersLib:InitialTransmittedTorqueNm_MP"
      mask help: physmod:simscape:couplers:SimscapeNetworkCouplersLib:NetworkCouplerFlexibleShaftPort1Interface_MD
      mask init:
      | % Fixed step sample time value check
      | foundation.internal.couplers.checkSampleTimes(gcb,h1,h2);
      | 
      | % Map mask choices to Simscape block parameters  
      | [K,Lambda,tau,~,~,x0,~] = foundation.internal.couplers.mechanical.derivedParamsRotational(...
      |     gcb,ts,h1,h2,through0,k,lambda,J1,J2);
      settings: PortSchema="{\"entries\":[{\"content\":{\"sides\":[{\"content\":{\"connectorIds\":[\"LConn1\"]},\"type\":\"ConnectorPlacement.EquallySpacedRectSide\",\"uuid\":\"a6d4a9fd-b5aa-40dc-ab7e-2b646b9b57bc\"},{\"content\":{\"connectorIds\":[\"Out1\",\"In1\"],\"side\":\"RIGHT\"},\"type\":\"ConnectorPlacement.EquallySpacedRectSide\",\"uuid\":\"31bb6273-5b9b-48d0-a1a2-6fbacb979b97\"},{\"content\":{\"connectorIds\":[],\"side\":\"TOP\"},\"type\":\"ConnectorPlacement.EquallySpacedRectSide\",\"uuid\":\"0f7afab2-4481-486c-9ad0-2b42c5b091a4\"}]},\"type\":\"ConnectorPlacement.EquallySpacedConnector\",\"uuid\":\"a98e47aa-cbfd-441a-b14c-c9ea515c056e\"}],\"packageUris\":[\"http://schema.mathworks.com/mf0/Connector/R2020b\"],\"version\":\"1.0\"}"
      mask Help: web([docroot '/simscape/ref/networkcouplerflexibleshaft.html'])
      mask TypeOptions interfaceModel: physmod:simscape:couplers:SimscapeNetworkCouplersLib:anActualShaftCompliance_PV | physmod:simscape:couplers:SimscapeNetworkCouplersLib:anAddedNumericalCompliance_PV
      mask Callback interfaceModel: foundation.internal.couplers.mechanical.parameterVisibilities(gcb)
      mask TypeOptions samplingType: physmod:simscape:couplers:SimscapeNetworkCouplersLib:VariableStepAtPorts1And2_PV | physmod:simscape:couplers:SimscapeNetworkCouplersLib:VariableStepAtPort1AndFixedStepAtPort2_PV | physmod:simscape:couplers:SimscapeNetworkCouplersLib:FixedStepBothPortsWithCommonSampleTime_PV | physmod:simscape:couplers:SimscapeNetworkCouplersLib:FixedStepBothPortsWithFasterSamplingAtPort1_PV
      mask Callback samplingType: foundation.internal.couplers.mechanical.parameterVisibilities(gcb)
      mask Callback predictionDiscreteToContinuous: foundation.internal.couplers.mechanical.parameterVisibilities(gcb)
      mask Callback smoothingContinuousToDiscrete: foundation.internal.couplers.mechanical.parameterVisibilities(gcb)
      mask Callback predictionSlowToFast: foundation.internal.couplers.mechanical.parameterVisibilities(gcb)
      mask Callback smoothingFastToSlow: foundation.internal.couplers.mechanical.parameterVisibilities(gcb)
      mask DialogControl Main Prompt: physmod:simscape:couplers:SimscapeNetworkCouplersLib:tab_Main
      mask DialogControl interfaceModel Prompt: Separate using
      mask DialogControl k Prompt: Shaft stiffness (Nm/rad)
      mask DialogControl lambda Prompt: Shaft damping (Nm/(rad/s))
      mask DialogControl samplingType Prompt: Sampling type
      mask DialogControl ts Prompt: Separator time constant (s)
      mask DialogControl h1 Prompt: Port 1 network discrete sample time (s)
      mask DialogControl h2 Prompt: Port 2 network discrete sample time (s)
      mask DialogControl predictionDiscreteToContinuous Prompt: Use prediction when connecting fixed step to variable step
      mask DialogControl smoothingContinuousToDiscrete Prompt: Use smoothing when connecting variable step to fixed step
      mask DialogControl predictionSlowToFast Prompt: Use prediction when connecting slow to fast sample times
      mask DialogControl smoothingFastToSlow Prompt: Use smoothing when connecting fast to slow sample times
      mask DialogControl nSmooth Prompt: Number of samples over which to smooth
      mask DialogControl tsSmoothing Prompt: Smoothing time constant (s)
      mask DialogControl Analysis Prompt: physmod:simscape:couplers:SimscapeNetworkCouplersLib:tab_Analysis
      mask DialogControl connectedNetworkInfo Prompt: physmod:simscape:couplers:SimscapeNetworkCouplersLib:heading_ConnectedNetworkInformation
      mask DialogControl J1 Prompt: Approximate inertia at port 1 (kg*m^2)
      mask DialogControl J2 Prompt: Approximate inertia at port 2 (kg*m^2)
      mask DialogControl derivedValues Prompt: physmod:simscape:couplers:SimscapeNetworkCouplersLib:heading_DerivedValues
      mask DialogControl tsRecommended Prompt: Recommended max filter time constant (s)
      mask DialogControl hRecommended Prompt: Recommended max discrete sample time (s)
      mask DialogControl kDerived Prompt: Calculated shaft stiffness (Nm/rad)
      mask DialogControl lambdaDerived Prompt: Calculated shaft damping (Nm/(rad/s))
      mask DialogControl tsMax Prompt: Calculated fastest trackable time constant (s)
      mask DialogControl updateRecommendations Prompt: physmod:simscape:couplers:SimscapeNetworkCouplersLib:button_Update
      mask DialogControl updateRecommendations Callback: foundation.internal.couplers.mechanical.analysisRotational(gcb);
      mask DialogControl InitialConditions Prompt: physmod:simscape:couplers:SimscapeNetworkCouplersLib:tab_InitialConditions
      mask DialogControl through0 Prompt: Initial transmitted torque (Nm)
  Rate transition (fast-to-slow) : RateTransition  Integrity=off  OutPortSampleTime=mbsTimeStep
  Scope : Scope  NumInputPorts=2
      settings: ActiveDisplayYMinimum=-4.84019  ActiveDisplayYMaximum=4.44418
  E : PMIOPort  Side=Left
  trq : Outport
  wires:
  First Order Hold3/1 -> Gain/1
  Port 1 Interface/1(torque) -> Gain1/1
  PS-Simulink Converter/1 -> Mux/1
  Mux/1 -> Scope/1
  Rate transition (fast-to-slow)/1 -> Scope/2, trq/1
  spd/1 -> First Order Hold3/1, Mux/2
  Gain/1 -> Port 1 Interface/1(speed)
  Gain1/1 -> Rate transition (fast-to-slow)/1
  connections:
  E/RConn1 -- Ideal Rotational Motion Sensor/LConn1 -- Port 1 Interface/LConn1
  PS-Simulink Converter/LConn1 -- Ideal Rotational Motion Sensor/RConn1

== system Excavator_Mevea_BucketDriveline/Excavator/Machine/Mevea/Interface CrawlerR ==
  note: Uncomment rate transition
      | blocks if one or both networks
      | are running fixed step.
  spd : Inport
  First Order Hold3 : FirstOrderHold  ErrorTolerance=inf  AllowContinuousInput=on
  Gain : Gain
  Gain1 : Gain  Gain=-1
  Ideal Rotational Motion Sensor : fl_lib/Mechanical/Mechanical Sensors/Ideal Rotational Motion Sensor  reference=foundation.enum.MeasurementReference.absolute  acceleration_port=false  velocity_port=true  position_port=false  wrap_angle=false  offset=0 rad
  Mux : Mux  Inputs=2
  PS-Simulink Converter : nesl_utility/PS-Simulink Converter  PhysicalDomain=network_engine_domain  SubClassName=ps_output  LeftPortType=input  RightPortType=output  PseudoPeriodic=off  Frequencies=[]  VectorFormat=inherit  Unit=rad/s  AffineConversion=off
  Port 1 Interface : Subsystem  mask(Network Coupler (Flexible Shaft) Port 1 Interface){interfaceModel=an actual shaft compliance, k=2500, lambda=200, samplingType=Variable step at ports 1 and 2, ts=0.002, h1=0.001, h2=0.01, predictionDiscreteToContinuous=off, smoothingContinuousToDiscrete=off, predictionSlowToFast=off, smoothingFastToSlow=off, nSmooth=1, tsSmoothing=0.01, J1=1, J2=1, tsRecommended=NaN, hRecommended=2.7764e-05, kDerived=2500, lambdaDerived=200, tsMax=0.012494, through0=0}
      mask prompts: interfaceModel "physmod:simscape:couplers:SimscapeNetworkCouplersLib:SeparateUsing_MP"; k "physmod:simscape:couplers:SimscapeNetworkCouplersLib:ShaftStiffnessNmrad_MP"; lambda "physmod:simscape:couplers:SimscapeNetworkCouplersLib:ShaftDampingNmrads_MP"; samplingType "physmod:simscape:couplers:SimscapeNetworkCouplersLib:SamplingType_MP"; ts "physmod:simscape:couplers:SimscapeNetworkCouplersLib:SeparatorTimeConstants_MP"; h1 "physmod:simscape:couplers:SimscapeNetworkCouplersLib:Port1NetworkDiscreteSampleTimes_MP"; h2 "physmod:simscape:couplers:SimscapeNetworkCouplersLib:Port2NetworkDiscreteSampleTimes_MP"; predictionDiscreteToContinuous "physmod:simscape:couplers:SimscapeNetworkCouplersLib:UsePredictionWhenConnectingFixedStepToVariableStep_MP"; smoothingContinuousToDiscrete "physmod:simscape:couplers:SimscapeNetworkCouplersLib:UseSmoothingWhenConnectingVariableStepToFixedStep_MP"; predictionSlowToFast "physmod:simscape:couplers:SimscapeNetworkCouplersLib:UsePredictionWhenConnectingSlowToFastSampleTimes_MP"; smoothingFastToSlow "physmod:simscape:couplers:SimscapeNetworkCouplersLib:UseSmoothingWhenConnectingFastToSlowSampleTimes_MP"; nSmooth "physmod:simscape:couplers:SimscapeNetworkCouplersLib:NumberOfSamplesOverWhichToSmooth_MP"; tsSmoothing "physmod:simscape:couplers:SimscapeNetworkCouplersLib:SmoothingTimeConstants_MP"; J1 "physmod:simscape:couplers:SimscapeNetworkCouplersLib:ApproximateInertiaAtPort1kgm2_MP"; J2 "physmod:simscape:couplers:SimscapeNetworkCouplersLib:ApproximateInertiaAtPort2kgm2_MP"; tsRecommended "physmod:simscape:couplers:SimscapeNetworkCouplersLib:RecommendedMaxFilterTimeConstants_MP"; hRecommended "physmod:simscape:couplers:SimscapeNetworkCouplersLib:RecommendedMaxDiscreteSampleTimes_MP"; kDerived "physmod:simscape:couplers:SimscapeNetworkCouplersLib:CalculatedShaftStiffnessNmrad_MP"; lambdaDerived "physmod:simscape:couplers:SimscapeNetworkCouplersLib:CalculatedShaftDampingNmrads_MP"; tsMax "physmod:simscape:couplers:SimscapeNetworkCouplersLib:CalculatedFastestTrackableTimeConstants_MP"; through0 "physmod:simscape:couplers:SimscapeNetworkCouplersLib:InitialTransmittedTorqueNm_MP"
      mask help: physmod:simscape:couplers:SimscapeNetworkCouplersLib:NetworkCouplerFlexibleShaftPort1Interface_MD
      mask init: same as Excavator_Mevea_BucketDriveline/Excavator/Machine/Mevea/Interface CrawlerL/Port 1 Interface
      settings: PortSchema="{\"entries\":[{\"content\":{\"sides\":[{\"content\":{\"connectorIds\":[\"LConn1\"]},\"type\":\"ConnectorPlacement.EquallySpacedRectSide\",\"uuid\":\"a6d4a9fd-b5aa-40dc-ab7e-2b646b9b57bc\"},{\"content\":{\"connectorIds\":[\"Out1\",\"In1\"],\"side\":\"RIGHT\"},\"type\":\"ConnectorPlacement.EquallySpacedRectSide\",\"uuid\":\"31bb6273-5b9b-48d0-a1a2-6fbacb979b97\"},{\"content\":{\"connectorIds\":[],\"side\":\"TOP\"},\"type\":\"ConnectorPlacement.EquallySpacedRectSide\",\"uuid\":\"0f7afab2-4481-486c-9ad0-2b42c5b091a4\"}]},\"type\":\"ConnectorPlacement.EquallySpacedConnector\",\"uuid\":\"a98e47aa-cbfd-441a-b14c-c9ea515c056e\"}],\"packageUris\":[\"http://schema.mathworks.com/mf0/Connector/R2020b\"],\"version\":\"1.0\"}"
      mask Help: web([docroot '/simscape/ref/networkcouplerflexibleshaft.html'])
      mask TypeOptions interfaceModel: physmod:simscape:couplers:SimscapeNetworkCouplersLib:anActualShaftCompliance_PV | physmod:simscape:couplers:SimscapeNetworkCouplersLib:anAddedNumericalCompliance_PV
      mask Callback interfaceModel: foundation.internal.couplers.mechanical.parameterVisibilities(gcb)
      mask TypeOptions samplingType: physmod:simscape:couplers:SimscapeNetworkCouplersLib:VariableStepAtPorts1And2_PV | physmod:simscape:couplers:SimscapeNetworkCouplersLib:VariableStepAtPort1AndFixedStepAtPort2_PV | physmod:simscape:couplers:SimscapeNetworkCouplersLib:FixedStepBothPortsWithCommonSampleTime_PV | physmod:simscape:couplers:SimscapeNetworkCouplersLib:FixedStepBothPortsWithFasterSamplingAtPort1_PV
      mask Callback samplingType: foundation.internal.couplers.mechanical.parameterVisibilities(gcb)
      mask Callback predictionDiscreteToContinuous: foundation.internal.couplers.mechanical.parameterVisibilities(gcb)
      mask Callback smoothingContinuousToDiscrete: foundation.internal.couplers.mechanical.parameterVisibilities(gcb)
      mask Callback predictionSlowToFast: foundation.internal.couplers.mechanical.parameterVisibilities(gcb)
      mask Callback smoothingFastToSlow: foundation.internal.couplers.mechanical.parameterVisibilities(gcb)
      mask DialogControl Main Prompt: physmod:simscape:couplers:SimscapeNetworkCouplersLib:tab_Main
      mask DialogControl interfaceModel Prompt: Separate using
      mask DialogControl k Prompt: Shaft stiffness (Nm/rad)
      mask DialogControl lambda Prompt: Shaft damping (Nm/(rad/s))
      mask DialogControl samplingType Prompt: Sampling type
      mask DialogControl ts Prompt: Separator time constant (s)
      mask DialogControl h1 Prompt: Port 1 network discrete sample time (s)
      mask DialogControl h2 Prompt: Port 2 network discrete sample time (s)
      mask DialogControl predictionDiscreteToContinuous Prompt: Use prediction when connecting fixed step to variable step
      mask DialogControl smoothingContinuousToDiscrete Prompt: Use smoothing when connecting variable step to fixed step
      mask DialogControl predictionSlowToFast Prompt: Use prediction when connecting slow to fast sample times
      mask DialogControl smoothingFastToSlow Prompt: Use smoothing when connecting fast to slow sample times
      mask DialogControl nSmooth Prompt: Number of samples over which to smooth
      mask DialogControl tsSmoothing Prompt: Smoothing time constant (s)
      mask DialogControl Analysis Prompt: physmod:simscape:couplers:SimscapeNetworkCouplersLib:tab_Analysis
      mask DialogControl connectedNetworkInfo Prompt: physmod:simscape:couplers:SimscapeNetworkCouplersLib:heading_ConnectedNetworkInformation
      mask DialogControl J1 Prompt: Approximate inertia at port 1 (kg*m^2)
      mask DialogControl J2 Prompt: Approximate inertia at port 2 (kg*m^2)
      mask DialogControl derivedValues Prompt: physmod:simscape:couplers:SimscapeNetworkCouplersLib:heading_DerivedValues
      mask DialogControl tsRecommended Prompt: Recommended max filter time constant (s)
      mask DialogControl hRecommended Prompt: Recommended max discrete sample time (s)
      mask DialogControl kDerived Prompt: Calculated shaft stiffness (Nm/rad)
      mask DialogControl lambdaDerived Prompt: Calculated shaft damping (Nm/(rad/s))
      mask DialogControl tsMax Prompt: Calculated fastest trackable time constant (s)
      mask DialogControl updateRecommendations Prompt: physmod:simscape:couplers:SimscapeNetworkCouplersLib:button_Update
      mask DialogControl updateRecommendations Callback: foundation.internal.couplers.mechanical.analysisRotational(gcb);
      mask DialogControl InitialConditions Prompt: physmod:simscape:couplers:SimscapeNetworkCouplersLib:tab_InitialConditions
      mask DialogControl through0 Prompt: Initial transmitted torque (Nm)
  Rate transition (fast-to-slow) : RateTransition  Integrity=off  OutPortSampleTime=mbsTimeStep
  Scope : Scope  NumInputPorts=2
      settings: ActiveDisplayYMinimum=-604.83961  ActiveDisplayYMaximum=604.8396
  E : PMIOPort  Side=Right
  trq : Outport
  wires:
  First Order Hold3/1 -> Gain/1
  Port 1 Interface/1(torque) -> Gain1/1
  PS-Simulink Converter/1 -> Mux/1
  Mux/1 -> Scope/1
  Rate transition (fast-to-slow)/1 -> Scope/2, trq/1
  spd/1 -> First Order Hold3/1, Mux/2
  Gain/1 -> Port 1 Interface/1(speed)
  Gain1/1 -> Rate transition (fast-to-slow)/1
  connections:
  E/RConn1 -- Ideal Rotational Motion Sensor/LConn1 -- Port 1 Interface/LConn1
  PS-Simulink Converter/LConn1 -- Ideal Rotational Motion Sensor/RConn1

== system Excavator_Mevea_BucketDriveline/Excavator/Machine/Mevea/Sensor Bucket ==
  Bucket Motion Sensor : Subsystem
  Demux1 : Demux  Outputs=3
  Demux2 : Demux  Outputs=3
  Demux3 : Demux  Outputs=3
  Demux4 : Demux
  Mux4 : Mux  Inputs=13
  Rate Transition{,1..3} (4 alike) : RateTransition  OutPortSampleTime=mbsTimeStep
  F : PMIOPort  Side=Left
  B : PMIOPort  Port=2  Side=Left
  m : Outport
  wires:
  Demux3/2 -> Mux4/5
  Demux2/2 -> Mux4/2
  Mux4/1 -> m/1
  Demux4/4 -> Mux4/13
  Demux4/2 -> Mux4/11
  Demux3/3 -> Mux4/6
  Demux1/3 -> Mux4/9
  Rate Transition2/1 -> Demux1/1
  Demux4/3 -> Mux4/12
  Rate Transition/1 -> Demux2/1
  Bucket Motion Sensor/4(quaternion) -> Rate Transition3/1
  Bucket Motion Sensor/2(angVel) -> Rate Transition1/1
  Demux4/1 -> Mux4/10
  Rate Transition1/1 -> Demux3/1
  Bucket Motion Sensor/1(vel) -> Rate Transition/1
  Rate Transition3/1 -> Demux4/1
  Demux1/1 -> Mux4/7
  Demux2/3 -> Mux4/3
  Bucket Motion Sensor/3(pos) -> Rate Transition2/1
  Demux3/1 -> Mux4/4
  Demux2/1 -> Mux4/1
  Demux1/2 -> Mux4/8
  connections:
  Bucket Motion Sensor/LConn1 -- F/RConn1
  B/RConn1 -- Bucket Motion Sensor/LConn2
